simulink model "H_inf_sim"  (R2022a)
settings: Solver=VariableStepAuto  StartTime=0.0  StopTime=10  RelTol=1e-3
undefined symbols (not defined in the file): A, B, C, D
libraries: cstblocks x3
settings Model: Creator=valen  LastModifiedBy=valen

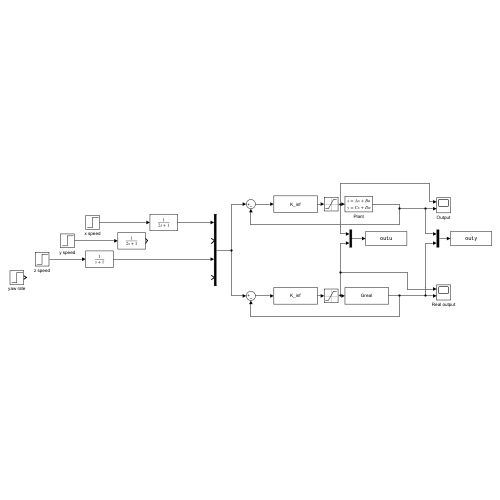
[thumbnail: Simulink's stored preview of the top-level diagram]
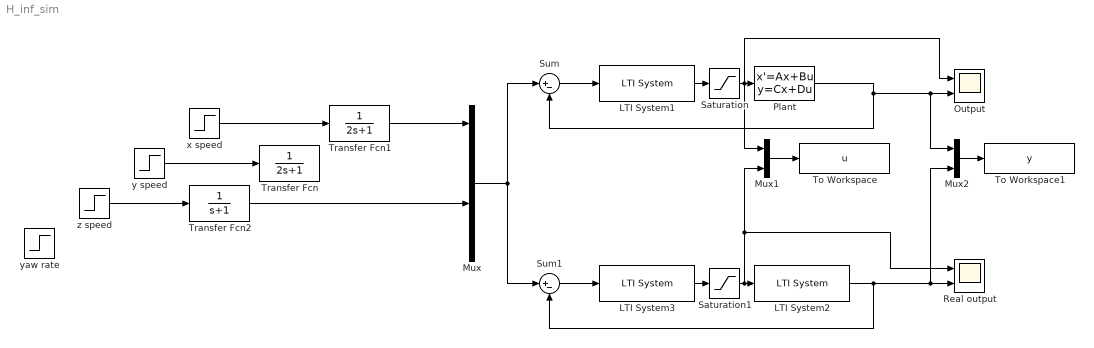
== system H_inf_sim ==
  LTI System1 : cstblocks/LTI System  sys=K_inf  IC=[]
  LTI System2 : cstblocks/LTI System  sys=Greal  IC=[]
  LTI System3 : cstblocks/LTI System  sys=K_inf  IC=[]
  Mux : Mux
  Mux1 : Mux  Inputs=2
  Mux2 : Mux  Inputs=2
  Output : Scope  NumInputPorts=2
  Plant : StateSpace  A=A  B=B  C=C  D=D  InitialCondition=0
  Real output : Scope  NumInputPorts=2
  Saturation : Saturate  UpperLimit=1  LowerLimit=-1
  Saturation1 : Saturate  UpperLimit=1  LowerLimit=-1
  Sum : Sum  Inputs=|+-
  Sum1 : Sum  Inputs=|+-
  To Workspace : ToWorkspace  VariableName=u  SaveFormat=Structure With Time  SampleTime=-1
  To Workspace1 : ToWorkspace  VariableName=y  SaveFormat=Structure With Time  SampleTime=-1
  Transfer Fcn : TransferFcn  Denominator=[2 1]
  Transfer Fcn1 : TransferFcn  Denominator=[2 1]
  Transfer Fcn2 : TransferFcn  Denominator=[1 1]
  x speed : Step  Time=0  SampleTime=0
  y speed : Step  Time=0  SampleTime=0
  yaw rate : Step  Time=0  SampleTime=0
  z speed : Step  Time=3  After=0.5  SampleTime=0
  wires:
  Sum/1 -> LTI System1/1
  Plant/1 -> Sum/2, Mux2/1, Output/2
  LTI System2/1 -> Mux2/2, Real output/2, Sum1/2
  Sum1/1 -> LTI System3/1
  Mux/1 -> Sum1/1, Sum/1
  y speed/1 -> Transfer Fcn/1
  x speed/1 -> Transfer Fcn1/1
  z speed/1 -> Transfer Fcn2/1
  Transfer Fcn1/1 -> Mux/1
  Transfer Fcn2/1 -> Mux/3
  LTI System1/1 -> Saturation/1
  Saturation/1 -> Output/1, Mux1/1, Plant/1
  LTI System3/1 -> Saturation1/1
  Saturation1/1 -> Real output/1, Mux1/2, LTI System2/1
  Mux1/1 -> To Workspace/1
  Mux2/1 -> To Workspace1/1
